simulink model "IFFLP_NON_LIN"  (R2021a)
settings: Solver=VariableStepAuto  StartTime=0.0  StopTime=150  RelTol=1e-3
model workspace (MATLAB code in the model file):
  | Kab=12;
  | Kcb=16;
  | Fb=4;
  | Kba=5;
  | Kca=8;
  | Kia=8;
  | Fa=6;
  | In=0.3;
  | x_star=[0.4;0.5;0.4];
settings Model: Creator=priya  LastModifiedBy=Priyan_PC
settings SolverCC: AlgebraicLoopSolver=TrustRegion
settings DebuggingCC: SFMachineParentedDataDiag=warning

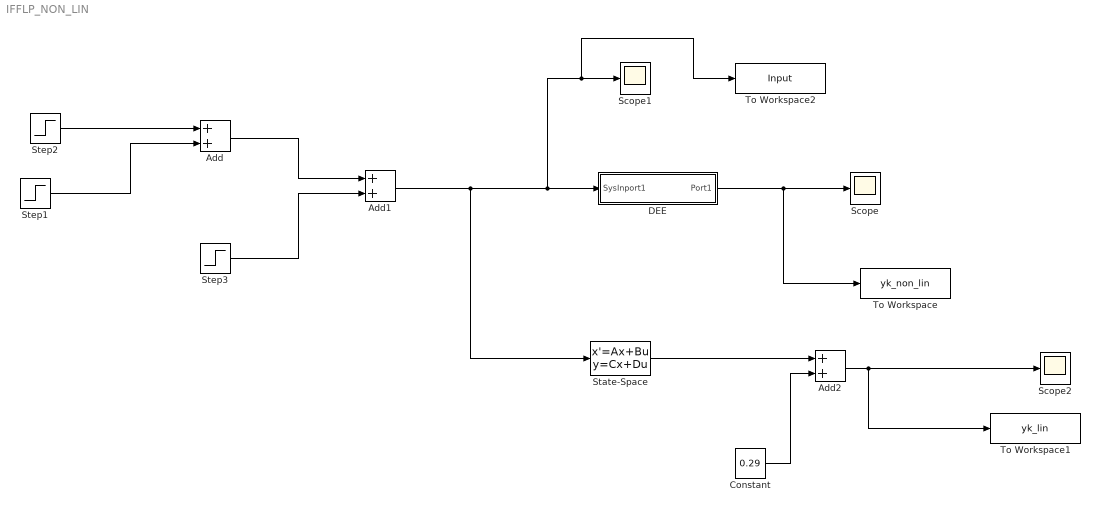
== system IFFLP_NON_LIN ==
  Add : Sum
  Add1 : Sum
  Add2 : Sum
  Constant : Constant  Value=0.29
  DEE : Subsystem  mask(Differential Equation Editor (DEE)){}
      settings: OpenFcn=diffeqed
      mask Display: disp('Differential Equation\n Editor')
  Scope : Scope
  Scope1 : Scope
  Scope2 : Scope
  State-Space : StateSpace  A=[-6 0 0;5 -4 0;8 -6.4 -8]  B=[8;0;0]  C=[0 0 1]  D=0  InitialCondition=0
  Step1 : Step  Time=15  After=0.15  SampleTime=0
  Step2 : Step  Time=0  Before=0.3  After=0.45  SampleTime=0
  Step3 : Step  Time=30  After=0.15  SampleTime=0
  To Workspace : ToWorkspace  VariableName=yk_non_lin  SampleTime=-1
  To Workspace1 : ToWorkspace  VariableName=yk_lin  SampleTime=-1
  To Workspace2 : ToWorkspace  VariableName=Input  SampleTime=-1
  wires:
  DEE/1(Port1) -> To Workspace/1, Scope/1
  Step2/1 -> Add/1
  Add1/1 -> State-Space/1, To Workspace2/1, Scope1/1, DEE/1(SysInport1)
  Step1/1 -> Add/2
  Add/1 -> Add1/1
  Step3/1 -> Add1/2
  State-Space/1 -> Add2/1
  Constant/1 -> Add2/2
  Add2/1 -> To Workspace1/1, Scope2/1

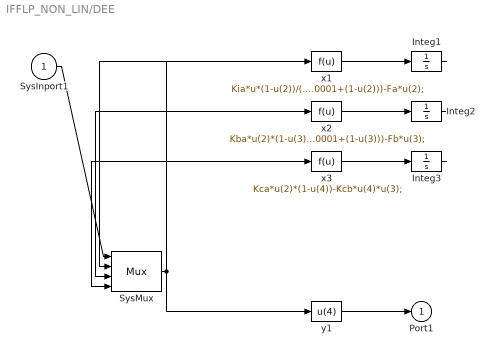
== system IFFLP_NON_LIN/DEE ==
  SysInport1 : Inport
  Integ1 : Integrator  InitialCondition=x_star(1)
  Integ2 : Integrator  InitialCondition=x_star(2)
  Integ3 : Integrator  InitialCondition=x_star(3)
  SysMux : Mux
  x1 : Fcn  Expr=Kia*u*(1-u(2))/(0.0001+(1-u(2)))-Fa*u(2);
  x2 : Fcn  Expr=Kba*u(2)*(1-u(3))/(0.00001+(1-u(3)))-Fb*u(3);
  x3 : Fcn  Expr=Kca*u(2)*(1-u(4))-Kcb*u(4)*u(3);
  y1 : Fcn  Expr=u(4)
  Port1 : Outport
  wires:
  SysInport1/1 -> SysMux/1
  SysMux/1 -> x1/1, x2/1, x3/1, y1/1
  x1/1 -> Integ1/1
  Integ1/1 -> SysMux/2
  x2/1 -> Integ2/1
  Integ2/1 -> SysMux/3
  x3/1 -> Integ3/1
  Integ3/1 -> SysMux/4
  y1/1 -> Port1/1
